simulink model "nxtReadData"  (R2014b)
settings: Solver=FixedStepDiscrete  StartTime=0.0  StopTime=inf  FixedStep=0.05  RelTol=1e-3
InitFcn:
  | nxt = comms.Bt(RobotID.NXT);
  | nxt.init();
  | nxt.reset();
  | nxt.init();
libraries: hostCommsLib x2, simulink x1, utility x1
settings Model: Creator=nrattner  LastModifiedBy=gatinc

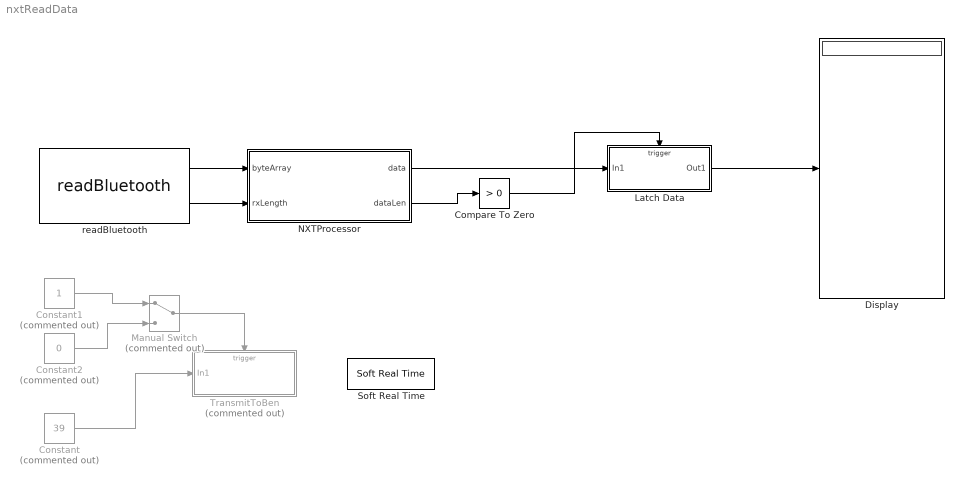
== system nxtReadData ==
  Compare To Zero : simulink/Logic and Bit Operations/Compare To Zero  relop=>  OutDataTypeStr=boolean
  Constant : Constant  Commented=on  Value=39
  Constant1 : Constant  Commented=on  SampleTime=-1
  Constant2 : Constant  Commented=on  Value=0  SampleTime=-1
  Display : Display
  Latch Data : Subsystem  TreatAsAtomicUnit=on
  Manual Switch : ManualSwitch  Commented=on
  NXTProcessor : MATLAB Function  TreatAsAtomicUnit=on
  Soft Real Time : utility/Soft Real Time  x=1
  TransmitToBen : Subsystem  Commented=on  TreatAsAtomicUnit=on
  readBluetooth : hostCommsLib/readBluetooth  robotId=RobotID.NXT  numBytes=4
  wires:
  Compare To Zero/1 -> Latch Data/Trigger
  Constant/1 -> TransmitToBen/1(In1)
  readBluetooth/2 -> NXTProcessor/2(rxLength)
  NXTProcessor/2(dataLen) -> Compare To Zero/1
  NXTProcessor/1(data) -> Latch Data/1(In1)
  Manual Switch/1 -> TransmitToBen/Trigger
  Constant1/1 -> Manual Switch/1
  Constant2/1 -> Manual Switch/2
  Latch Data/1(Out1) -> Display/1
  readBluetooth/1 -> NXTProcessor/1(byteArray)

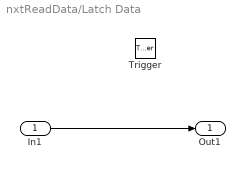
== system nxtReadData/Latch Data ==
  In1 : Inport
  Trigger : TriggerPort
  Out1 : Outport
  wires:
  In1/1 -> Out1/1

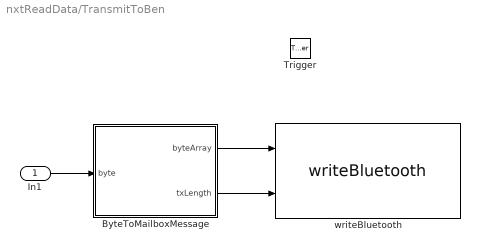
== system nxtReadData/TransmitToBen ==
  In1 : Inport
  Trigger : TriggerPort  TriggerType=either
  ByteToMailboxMessage : MATLAB Function  TreatAsAtomicUnit=on
  writeBluetooth : hostCommsLib/writeBluetooth  robotId=RobotID.NXT_BEN
  wires:
  In1/1 -> ByteToMailboxMessage/1(byte)
  ByteToMailboxMessage/1(byteArray) -> writeBluetooth/1
  ByteToMailboxMessage/2(txLength) -> writeBluetooth/2

== matlab function nxtReadData/TransmitToBen/ByteToMailboxMessage ==
  data: byte input; byteArray output; txLength output
function [byteArray,txLength] = fcn(byte)
%#codegen

byteArray = uint8([2 0 1 byte]);
txLength = 4;

== matlab function nxtReadData/NXTProcessor ==
  data: data output; dataLen output; byteArray input uint8; rxLength input double
function [data,dataLen] = nxtProcessor(byteArray,rxLength)
%#codegen

persistent ben;

if(isempty(ben))
    bufferLen = uint8(8);
    ben = comms.RawNXTDataProcessor(bufferLen);
end

[data,dataLen] = ben.process(byteArray,uint8(rxLength));

end
